simulink model "postlab"  (R2025b)
settings: Solver=VariableStepAuto  StartTime=0.0  StopTime=3  RelTol=1e-3
settings Model: Creator=Murl0  LastModifiedBy=Murl0

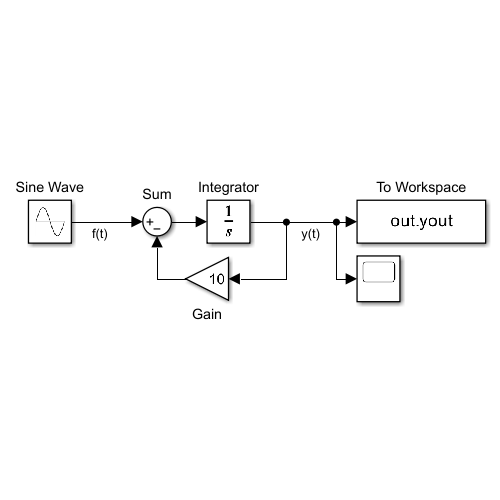
[thumbnail: Simulink's stored preview of the top-level diagram]
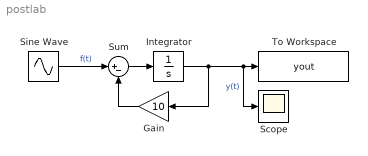
== system postlab ==
  Gain : Gain  Gain=10
  Integrator : Integrator  InitialCondition=1
  Scope : Scope
      settings: ActiveDisplayYMinimum=-0.33388046390907522  ActiveDisplayYMaximum=1.1482089404343416
  Sine Wave : Sin  Amplitude=2  Frequency=4  SampleTime=0
  Sum : Sum  Inputs=|+-
  To Workspace : ToWorkspace  VariableName=yout  SaveFormat=Timeseries  SampleTime=-1
  wires:
  Sine Wave/1 -> Sum/1  "f(t)"
  Sum/1 -> Integrator/1
  Integrator/1 -> Gain/1, Scope/1, To Workspace/1  "y(t)"
  Gain/1 -> Sum/2
